simulink model "Virtual_Exhaust_Aftertreatment_Controller_PRT"  (R2016b)
settings: Solver=FixedStepAuto  StartTime=0.0  StopTime=inf  FixedStep=VirtExhATCtrlr.tiSimnTiStep_C  RelTol=1e-3  SampleTimeConstraint=STIndependent  EnableMultiTasking=on
undefined symbols (not defined in the file or in its folder): CAL, SOUIT, T3LIMCL_COEOM_MSK_SY, T3LimCL_stMskEOM1_C, T3LimCL_stMskEOM2_C, T3LimCL_stMskEOM3_C, VirtExhATCtrlr_numHrznSize_CA
libraries: simulink x4
(part 5 of 5)

== system Virtual_Exhaust_Aftertreatment_Controller_PRT/UCatCtrl/Urea_Dosing_Control/Feedback Control/PIDctrl/SAT2 ==
  up : Inport
  u : Inport  Port=2
  lo : Inport  Port=3
  Data Type Duplicate : DataTypeDuplicate  DisableCoverage=on
  Data Type Propagation : S-Function  FunctionName=sfix_dtprop  Parameters=14,PropDataTypeMode,(getdatatypespecs(PropDataType,PropScaling,DblOver,0, 0, PropDataTypeMode, PropScalingMode)),IfRefDouble,IfRefSingle,IsSigned,NumBitsBase,NumBitsMult,NumBitsAdd,(sort(reshape(round(NumBitsAllowFinal), prod(size(NumBitsAllowFinal)),1))),PropScalingMode,ValuesUsedBestPrec,SlopeBase,SlopeMult,SlopeAdd,BiasBase,BiasMult,BiasAdd,DblOver  SFunctionDeploymentMode=off  EnableBusSupport=off  mask(Data Type Propagation){PropDataTypeMode=Inherit via propagation rule, PropDataType=fixdt(1, 16), IfRefDouble=double, IfRefSingle=single, IsSigned=IsSigned1, NumBitsBase=NumBits1, NumBitsMult=1, NumBitsAdd=0, NumBitsAllowFinal=1:128, PropScalingMode=Inherit via propagation rule, PropScaling=2^-10, ValuesUsedBestPrec=[5 -7], SlopeBase=Slope1, SlopeMult=1, SlopeAdd=0, BiasBase=Bias1, BiasMult=1, BiasAdd=0}
      mask prompts: PropDataTypeMode "Simulink:masks:x1PropagatedDataType_MP"; PropDataType "Simulink:masks:x11PropagatedDataTypeegFixdt116Fixdtsingle_MP"; IfRefDouble "Simulink:masks:x11IfAnyReferenceInputIsDoubleOutputIs_MP"; IfRefSingle "Simulink:masks:x12IfAnyReferenceInputIsSingleOutputIs_MP"; IsSigned "Simulink:masks:x13IsSigned_MP"; NumBitsBase "Simulink:masks:x141NumberofBitsBase_MP"; NumBitsMult "Simulink:masks:x142NumberofBitsMultiplicativeAdjustment_MP"; NumBitsAdd "Simulink:masks:x143NumberofBitsAdditiveAdjustment_MP"; NumBitsAllowFinal "Simulink:masks:x144NumberofBitsAllowableFinalValues_MP"; PropScalingMode "Simulink:masks:x2PropagatedScaling_MP"; PropScaling "Simulink:masks:x21PropagatedScalingSlopeEg29OrSlopeBiasEg1253_MP"; ValuesUsedBestPrec "Simulink:masks:x21ValuesUsedToDetermineBestPrecisionScaling_MP"; SlopeBase "Simulink:masks:x211SlopeBase_MP"; SlopeMult "Simulink:masks:x212SlopeMultiplicativeAdjustment_MP"; SlopeAdd "Simulink:masks:x213SlopeAdditiveAdjustment_MP"; BiasBase "Simulink:masks:x221BiasBase_MP"; BiasMult "Simulink:masks:x222BiasMultiplicativeAdjustment_MP"; BiasAdd "Simulink:masks:x223BiasAdditiveAdjustment_MP"
      mask help: Simulink:masks:DataTypePropagation_MD
      mask init:
      | DblOver = 0;
      mask TypeOptions PropDataTypeMode: Simulink:masks:SpecifyViaDialog | Simulink:masks:InheritViaPropagationRule
      mask Callback PropDataTypeMode: fixptdialog(gcbh)
      mask Callback PropDataType: fixptdialog(gcbh)
      mask TypeOptions IfRefDouble: Simulink:masks:double | Simulink:masks:single
      mask TypeOptions IfRefSingle: Simulink:masks:double | Simulink:masks:single
      mask TypeOptions IsSigned: Simulink:masks:IsSigned1 | Simulink:masks:IsSigned2 | Simulink:masks:IsSigned1OrIsSigned2 | Simulink:masks:TRUE | Simulink:masks:FALSE
      mask TypeOptions NumBitsBase: NumBits1 | NumBits2 | max([NumBits1 NumBits2]) | min([NumBits1 NumBits2]) | NumBits1+NumBits2
      mask TypeOptions PropScalingMode: Simulink:masks:SpecifyViaDialog | Simulink:masks:InheritViaPropagationRule | Simulink:masks:ObtainViaBestPrecision
      mask Callback PropScalingMode: fixptdialog(gcbh)
      mask TypeOptions SlopeBase: Slope1 | Slope2 | max([Slope1 Slope2]) | min([Slope1 Slope2]) | Slope1*Slope2 | Slope1/Slope2 | PosRange1 | PosRange2 | max([PosRange1 PosRange2]) | min([PosRange1 PosRange2]) | PosRange1*PosRange2 | PosRange1/PosRange2
      mask TypeOptions BiasBase: Bias1 | Bias2 | max([Bias1 Bias2]) | min([Bias1 Bias2]) | Bias1*Bias2 | Bias1/Bias2 | Bias1+Bias2 | Bias1-Bias2
      mask Display:
      | port_label('Input',1,'Ref1');
      | port_label('Input',2,'Ref2');
      | port_label('Input',3,'Prop');
  LowerRelop1 : RelationalOperator  DisableCoverage=on  Operator=>  OutDataTypeStr=boolean  RndMeth=Nearest
  Switch : Switch  Criteria=u2 ~= 0  OutDataTypeStr=Inherit: Inherit via back propagation  ZeroCross=off
  Switch2 : Switch  Criteria=u2 ~= 0  OutMin=OutMin  OutMax=OutMax  OutDataTypeStr=Inherit: Inherit via back propagation  ZeroCross=off
  UpperRelop : RelationalOperator  DisableCoverage=on  Operator=<  OutDataTypeStr=boolean  RndMeth=Nearest
  y : Outport  OutMin=OutMin  OutMax=OutMax
  wires:
  up/1 -> Switch2/1, LowerRelop1/2
  u/1 -> Data Type Propagation/2, Data Type Propagation/1, LowerRelop1/1, Switch/3, UpperRelop/1
  lo/1 -> Switch/1, UpperRelop/2
  Switch/1 -> Data Type Duplicate/2, Switch2/3, Data Type Propagation/3
  Switch2/1 -> Data Type Duplicate/1, y/1
  LowerRelop1/1 -> Switch2/2
  UpperRelop/1 -> Switch/2

== system Virtual_Exhaust_Aftertreatment_Controller_PRT/UCatCtrl/Urea_Dosing_Control/Feedback Control/PIDctrl/Subsystem ==
  X : Inport
  Ki : Inport  Port=2
  Reset : Inport  Port=3
  Y0_YReset : Inport  Port=4
  Min : Inport  Port=5
  Max : Inport  Port=6
  dT : Inport  Port=7
  Add1 : Sum
  Add2 : Sum
  AntiWindUp : Subsystem
  Constant2 : Constant  Value=0  SampleTime=-1
  Constant3 : Constant  Value=0  SampleTime=-1
  Kp = 0 : Constant  Value=0  SampleTime=-1
  Product1 : Product  RndMeth=Zero
  Product2 : Product  RndMeth=Zero
  Product3 : Product  RndMeth=Zero
  Saturation : Subsystem
  Switch1 : Switch  Criteria=u2 ~= 0
  Switch2 : Switch  Criteria=u2 ~= 0
  Switch3 : Switch  Criteria=u2 ~= 0
  Unit Delay External IC : Subsystem  mask(Unit Delay External Initial Condition){tsamp=-1}
      mask prompts: tsamp "Simulink:masks:SampleTime_MP"
      mask help: Simulink:masks:UnitDelayExternalInitialCondition_MD
      mask Display: dpoly(1,[1 0],'z')
  Unit Delay External IC1 : Subsystem  mask(Unit Delay External Initial Condition){tsamp=-1}
      mask prompts: tsamp "Simulink:masks:SampleTime_MP"
      mask help: Simulink:masks:UnitDelayExternalInitialCondition_MD
      mask Display: dpoly(1,[1 0],'z')
  Y : Outport
  wires:
  Constant3/1 -> Switch3/1
  AntiWindUp/1(Clamp) -> Switch1/2
  Saturation/1(Y) -> Unit Delay External IC1/1(u)
  Product1/1 -> Switch3/3
  Product2/1 -> Product3/1
  Product3/1 -> AntiWindUp/1(PreInteg), Switch1/3
  Add1/1 -> Switch2/3
  Saturation/2(Sat) -> AntiWindUp/2(Sat)
  Switch1/1 -> Add1/1
  Switch3/1 -> Add2/1
  Add2/1 -> Saturation/2(X)
  Switch2/1 -> Add2/2, Unit Delay External IC/1(u)
  Reset/1 -> Switch2/2, Switch3/2
  X/1 -> Product2/1, Product1/1
  Max/1 -> Saturation/1(Max)
  Y0_YReset/1 -> Switch2/1, Unit Delay External IC/2(IC), Unit Delay External IC1/2(IC)
  Unit Delay External IC1/1(y) -> Y/1
  dT/1 -> Product3/2
  Unit Delay External IC/1(y) -> Add1/2
  Ki/1 -> Product2/2
  Min/1 -> Saturation/3(Min)
  Kp = 0/1 -> Product1/2
  Constant2/1 -> Switch1/1

== system Virtual_Exhaust_Aftertreatment_Controller_PRT/UCatCtrl/Urea_Dosing_Control/Feedback Control/PIDctrl/Subsystem1 ==
  note: ( U(k) - U(k-1) )
  note: U(k)
  X : Inport
  Y0 : Inport  Port=2
  dT : Inport  Port=3
  Divide : Product  Inputs=*/
  Subtract : Sum  Inputs=+-
  Unit Delay External IC : Subsystem  mask(Unit Delay External Initial Condition){tsamp=-1}
      mask prompts: tsamp "Simulink:masks:SampleTime_MP"
      mask help: Simulink:masks:UnitDelayExternalInitialCondition_MD
      mask Display: dpoly(1,[1 0],'z')
  Y : Outport
  wires:
  X/1 -> Divide/1
  Divide/1 -> Subtract/1, Unit Delay External IC/1(u)
  dT/1 -> Divide/2
  Subtract/1 -> Y/1
  Unit Delay External IC/1(y) -> Subtract/2  "U(k-1)"
  Y0/1 -> Unit Delay External IC/2(IC)  "XX"

== system Virtual_Exhaust_Aftertreatment_Controller_PRT/UCatCtrl/Urea_Dosing_Control/Feedback Control/PIDctrl/Subsystem2 ==
  X : Inport
  Ki : Inport  Port=2
  Reset : Inport  Port=3
  Y0_YReset : Inport  Port=4
  Min : Inport  Port=5
  Max : Inport  Port=6
  dT : Inport  Port=7
  Add1 : Sum
  Add2 : Sum
  AntiWindUp : Subsystem
  Constant2 : Constant  Value=0  SampleTime=-1
  Constant3 : Constant  Value=0  SampleTime=-1
  Kp = 0 : Constant  Value=0  SampleTime=-1
  Product1 : Product  RndMeth=Zero
  Product2 : Product  RndMeth=Zero
  Product3 : Product  RndMeth=Zero
  Saturation : Subsystem
  Switch1 : Switch  Criteria=u2 ~= 0
  Switch2 : Switch  Criteria=u2 ~= 0
  Switch3 : Switch  Criteria=u2 ~= 0
  Unit Delay External IC : Subsystem  mask(Unit Delay External Initial Condition){tsamp=-1}
      mask prompts: tsamp "Simulink:masks:SampleTime_MP"
      mask help: Simulink:masks:UnitDelayExternalInitialCondition_MD
      mask Display: dpoly(1,[1 0],'z')
  Unit Delay External IC1 : Subsystem  mask(Unit Delay External Initial Condition){tsamp=-1}
      mask prompts: tsamp "Simulink:masks:SampleTime_MP"
      mask help: Simulink:masks:UnitDelayExternalInitialCondition_MD
      mask Display: dpoly(1,[1 0],'z')
  Y : Outport
  wires:
  Constant2/1 -> Switch1/1
  Kp = 0/1 -> Product1/2
  Min/1 -> Saturation/3(Min)
  Ki/1 -> Product2/2
  Unit Delay External IC/1(y) -> Add1/2
  dT/1 -> Product3/2
  Unit Delay External IC1/1(y) -> Y/1
  Y0_YReset/1 -> Unit Delay External IC1/2(IC), Unit Delay External IC/2(IC), Switch2/1
  Max/1 -> Saturation/1(Max)
  X/1 -> Product1/1, Product2/1
  Reset/1 -> Switch3/2, Switch2/2
  Switch2/1 -> Unit Delay External IC/1(u), Add2/2
  Add2/1 -> Saturation/2(X)
  Switch3/1 -> Add2/1
  Switch1/1 -> Add1/1
  Saturation/2(Sat) -> AntiWindUp/2(Sat)
  Add1/1 -> Switch2/3
  Product3/1 -> Switch1/3, AntiWindUp/1(PreInteg)
  Product2/1 -> Product3/1
  Product1/1 -> Switch3/3
  Saturation/1(Y) -> Unit Delay External IC1/1(u)
  AntiWindUp/1(Clamp) -> Switch1/2
  Constant3/1 -> Switch3/1

== system Virtual_Exhaust_Aftertreatment_Controller_PRT/UCatCtrl/SCR_Prediction/Main/UCat NH3 Load Prediction/Discrete Integrator/AntiWindUp ==
  PreInteg : Inport
  Sat : Inport  Port=2
  Constant1 : Constant  Value=0  SampleTime=-1
  Logical1 : Logic  AllPortsSameDT=off  OutDataTypeStr=boolean
  Relational1 : RelationalOperator  Operator===  OutDataTypeStr=boolean  RndMeth=Nearest
  Relational2 : RelationalOperator  Operator=~=  OutDataTypeStr=boolean  RndMeth=Nearest
  Sign1 : Signum
  UnitDelay2 : UnitDelay  SampleTime=-1
  Clamp : Outport
  wires:
  PreInteg/1 -> Sign1/1
  Sign1/1 -> Relational1/1
  Relational1/1 -> Logical1/1
  Sat/1 -> UnitDelay2/1
  Logical1/1 -> Clamp/1
  UnitDelay2/1 -> Relational2/1, Relational1/2
  Relational2/1 -> Logical1/2
  Constant1/1 -> Relational2/2

== system Virtual_Exhaust_Aftertreatment_Controller_PRT/UCatCtrl/SCR_Prediction/Main/UCat NH3 Load Prediction/Discrete Integrator/Saturation ==
  Max : Inport
  X : Inport  Port=2
  Min : Inport  Port=3
  Constant1 : Constant  SampleTime=-1
  Constant2 : Constant  Value=-1  SampleTime=-1
  Constant3 : Constant  Value=0  SampleTime=-1
  Relational1 : RelationalOperator  Operator=<  OutDataTypeStr=boolean  RndMeth=Nearest
  Relational2 : RelationalOperator  Operator=>  OutDataTypeStr=boolean  RndMeth=Nearest
  Switch{1..4} (4 alike) : Switch  Criteria=u2 ~= 0
  Y : Outport
  Sat : Outport  Port=2
  wires:
  Relational1/1 -> Switch4/2, Switch2/2
  Max/1 -> Switch2/1, Relational1/1
  Relational2/1 -> Switch3/2, Switch1/2
  Min/1 -> Relational2/1, Switch1/1
  Switch1/1 -> Switch2/3
  X/1 -> Relational1/2, Relational2/2, Switch1/3
  Switch2/1 -> Y/1
  Constant1/1 -> Switch4/1
  Switch3/1 -> Switch4/3
  Switch4/1 -> Sat/1
  Constant2/1 -> Switch3/1
  Constant3/1 -> Switch3/3

== system Virtual_Exhaust_Aftertreatment_Controller_PRT/UCatCtrl/SCR_Prediction/Main/UCat NH3 Load Prediction/Discrete Integrator/Unit Delay External IC ==
  note: Xnew
  note: Initial Value
  u : Inport
  IC : Inport  Port=2
  FixPt Constant : Constant  DisableCoverage=on  Value=0  OutDataTypeStr=fixdt(0,8,0)  SampleTime=-1
  FixPt Data Type Duplicate1 : DataTypeDuplicate  DisableCoverage=on  NumInputPorts=3
  FixPt Unit Delay1 : UnitDelay  DisableCoverage=on  InitialCondition=0.0  SampleTime=tsamp  HasFrameUpgradeWarning=off
  FixPt Unit Delay2 : UnitDelay  DisableCoverage=on  InitialCondition=1  SampleTime=tsamp
  Init : Switch  Criteria=u2 ~= 0  OutDataTypeStr=Inherit: Inherit via back propagation  ZeroCross=off
  y : Outport
  wires:
  FixPt Unit Delay1/1 -> Init/3  "Xold"
  Init/1 -> y/1, FixPt Data Type Duplicate1/1
  FixPt Unit Delay2/1 -> Init/2
  FixPt Constant/1 -> FixPt Unit Delay2/1
  u/1 -> FixPt Unit Delay1/1, FixPt Data Type Duplicate1/2
  IC/1 -> Init/1, FixPt Data Type Duplicate1/3

== system Virtual_Exhaust_Aftertreatment_Controller_PRT/UCatCtrl/SCR_Prediction/Main/UCat NH3 Load Prediction/Discrete Integrator/Unit Delay External IC1 ==
  note: Xnew
  note: Initial Value
  u : Inport
  IC : Inport  Port=2
  FixPt Constant : Constant  DisableCoverage=on  Value=0  OutDataTypeStr=fixdt(0,8,0)  SampleTime=-1
  FixPt Data Type Duplicate1 : DataTypeDuplicate  DisableCoverage=on  NumInputPorts=3
  FixPt Unit Delay1 : UnitDelay  DisableCoverage=on  InitialCondition=0.0  SampleTime=tsamp  HasFrameUpgradeWarning=off
  FixPt Unit Delay2 : UnitDelay  DisableCoverage=on  InitialCondition=1  SampleTime=tsamp
  Init : Switch  Criteria=u2 ~= 0  OutDataTypeStr=Inherit: Inherit via back propagation  ZeroCross=off
  y : Outport
  wires:
  FixPt Unit Delay1/1 -> Init/3  "Xold"
  Init/1 -> y/1, FixPt Data Type Duplicate1/1
  FixPt Unit Delay2/1 -> Init/2
  FixPt Constant/1 -> FixPt Unit Delay2/1
  u/1 -> FixPt Unit Delay1/1, FixPt Data Type Duplicate1/2
  IC/1 -> Init/1, FixPt Data Type Duplicate1/3

== system Virtual_Exhaust_Aftertreatment_Controller_PRT/UCatCtrl/SCR_Prediction/Main/UCat NH3 Load Prediction/GOTO_ATS_mflNH3OxiUCatUs_mgps/GainXX ==
  In : Inport
  Out : Outport
  wires:
  In/1 -> Out/1

== system Virtual_Exhaust_Aftertreatment_Controller_PRT/UCatCtrl/SCR_Prediction/Main/UCat NH3 Load Prediction/NH3 Oxidation/NH3 Oxidation ==
  ATS_mEstNH3LdUCat : Inport
  ATS_tEstUCatAvrg : Inport  Port=2
  ATS_rNH3Curr_ppm : Inport  Port=3
  "ATS_mflEG " : Inport  Port=4
  ATS_facEffUCatAge : Inport  Port=5
  Constant1 : Constant  Value=1000  SampleTime=-1
  Constant2 : Constant  Value=0  SampleTime=-1
  Constant6 : Constant  SampleTime=-1
  Lookup_n-D_3 : Lookup_n-D  BreakpointsForDimension1=[100;150;200;250;300;350;400;450;500;550;700;1000]  BreakpointsForDimension2=[0 1.89999997615814 3.79999995231628 5.69999980926514 7.59999990463257 11.3999996185303 15.1999998092651 26.6000003814697]  Table=[0 3.70879998570075e-20 7.42519969327932e-20 1.10959997771212e-19 1.48200004990473e-19 2.22679993579601e-19 2.97160008018124e-19 5.19840001597725e-19;0 9.04399990686384e-18 1.81639995140478e-17 2.72839999484124e-17 3.6404000382777e-17 5.45679998968249e-17 7.28080007655541e-17 1.26919999151736e-16;0 6.97680021648363e-16 1.39840004454442e-15 2.09000001075784e-15 2.78920008596961e-15 4.18760002463491e-15 5.57840017193921e-15 9.72799975746145e-15;0 2.3332000258702e-14 4.66640005174039e-14 6.99959973879741e-14 9.34799994031267e-14 1.39840003183893e-13 1.86200000188395e-13 3.26040003372288e-13;0 4.22559990470584e-13 8.43599983705451e-13 1.26920002285758e-12 1.6871999674109e-12 2.53840004571515e-12 3.38199997521049e-12 5.91280019737739e-12;0 4.81080019570923e-12 9.57599971540546e-12 1.43639995731082e-11 1.92279994010169e-11 2.88040008511459e-11 3.84559988020339e-11 6.73359978886623e-11;0 3.81519989212098e-11 7.59999979615955e-11 1.13999996942393e-10 1.51999995923191e-10 2.28759997056294e-10 3.04759995017889e-10 5.33520005951971e-10;0 2.2648000141956e-10 4.53720006010627e-10 6.80960010601694e-10 9.04399999335226e-10 1.36040001486038e-09 1.81640003038552e-09 3.17679993422359e-09;0 1.07160003093298e-09 2.14320006186597e-09 3.22239990246942e-09 4.2939998223801e-09 6.43720010629067e-09 8.5879996447602e-09 1.49720005282461e-08;0 4.20279988588845e-09 8.35999980353108e-09 1.26159998004027e-08 1.67959992580791e-08 2.52319996008055e-08 3.35919985161581e-08 5.88239998933204e-08;0 1.08679998334083e-07 2.16600000157996e-07 3.25280012702933e-07 4.3471999333633e-07 6.51320021916035e-07 8.66400000631984e-07 1.51999995523511e-06;0 7.28080021872302e-06 1.45920002978528e-05 2.18120003410149e-05 2.91079995804466e-05 4.37000016972888e-05 5.82159991608933e-05 0.000101839999842923]  ExtrapMethod=Clip  UseLastTableValue=on  RndMeth=Simplest  InputSameDT=on
  Lookup_n-D_4 : Lookup_n-D  BreakpointsForDimension1=[0;0.100000001490116;0.200000002980232;0.300000011920929;0.5;0.75;1]  BreakpointsForDimension2=[0 500 1000 1500 2000 2500 3000]  Table=[0.184162065386772 0.184162065386772 0.184162065386772 0.184162065386772 0.184162065386772 0.184162065386772 0.184162065386772;0.184162065386772 0.184162065386772 0.184162065386772 0.184162065386772 0.184162065386772 0.184162065386772 0.184162065386772;0.184162065386772 0.184162065386772 0.184162065386772 0.184162065386772 0.184162065386772 0.184162065386772 0.184162065386772;0.184162065386772 0.184162065386772 0.184162065386772 0.184162065386772 0.184162065386772 0.184162065386772 0.184162065386772;0.184162065386772 0.184162065386772 0.184162065386772 0.184162065386772 0.184162065386772 0.184162065386772 0.184162065386772;0.184162065386772 0.184162065386772 0.184162065386772 0.184162065386772 0.184162065386772 0.184162065386772 0.184162065386772;0.184162065386772 0.184162065386772 0.184162065386772 0.184162065386772 0.184162065386772 0.184162065386772 0.184162065386772]  RndMeth=Simplest  InputSameDT=on
  Lookup_n-D_5 : Lookup_n-D  BreakpointsForDimension1=[100;150;200;250;300;350;400;450;500;550;700;1000]  BreakpointsForDimension2=[0 75 175 350 550 1000]  Table=[10000000000 10000000000 10000000000 10000000000 10000000000 10000000000;10000000000 10000000000 10000000000 10000000000 10000000000 10000000000;10000000000 10000000000 10000000000 10000000000 10000000000 10000000000;2000000000 2000000000 4499999744 5470000128 12199999488 12199999488;600000000 600000000 1500000000 3100000000 4600000000 4600000000;120000000 120000000 200000000 300000000 450000000 500000000;25000000 25000000 32500000 49000000 51500000 51500000;12000000 12000000 20000000 30000000 38000000 38000000;3500000 3500000 6000000 11500000 14000000 14000000;2500000 2500000 5500000 8500000 10000000 10000000;2000000 2000000 4000000 5000000 8000000 8000000;1000000 1000000 2000000 3000000 5900000 5000000]  RndMeth=Simplest  InputSameDT=on
  Lookup_n-D_6 : Lookup_n-D  Description=output: mg/s  BreakpointsForDimension1=[0;0.100000001490116;0.200000002980232;0.300000011920929;0.5;0.75;1]  BreakpointsForDimension2=[0 500 1000 1500 2000 2500 3000]  Table=[1 1 1 1 1 1 1;1 1 1 1 1 1 1;1 1 1 1 1 1 1;1 1 1 1 1 1 1;1 1 1 1 1 1 1;1 1 1 1 1 1 1;1 1 1 1 1 1 1]  ExtrapMethod=Clip  UseLastTableValue=on  RndMeth=Simplest  InputSameDT=on
  MinMax : MinMax  Function=max  Inputs=2
  rox_gps{,1..3} (4 alike) : Product  SaturateOnIntegerOverflow=on  OutDataTypeStr=Inherit: Same as first input
  ATS_mflNH3OxiUCatUs_mgps : Outport
  wires:
  Lookup_n-D_5/1 -> rox_gps/2
  MinMax/1 -> rox_gps/1
  Constant2/1 -> MinMax/1
  ATS_rNH3Curr_ppm/1 -> Lookup_n-D_5/2
  Lookup_n-D_3/1 -> MinMax/2
  ATS_mEstNH3LdUCat/1 -> Lookup_n-D_3/2
  ATS_tEstUCatAvrg/1 -> Lookup_n-D_3/1, Lookup_n-D_5/1
  rox_gps1/1 -> rox_gps2/1
  Lookup_n-D_4/1 -> rox_gps1/2
  ATS_facEffUCatAge/1 -> Lookup_n-D_4/1
  "ATS_mflEG "/1 -> Lookup_n-D_6/2, Lookup_n-D_4/2
  rox_gps/1 -> rox_gps3/1
  Constant6/1 -> Lookup_n-D_6/1
  Lookup_n-D_6/1 -> rox_gps2/2
  rox_gps2/1 -> ATS_mflNH3OxiUCatUs_mgps/1
  Constant1/1 -> rox_gps3/2
  rox_gps3/1 -> rox_gps1/1

== system Virtual_Exhaust_Aftertreatment_Controller_PRT/UCatCtrl/SCR_Prediction/Main/UCat NH3 Load Prediction/NH3 Oxidation/mg//s to ppm ==
  ATS_mflNH3MetAdapDes_mgps : Inport
  ATS_mflEG : Inport  Port=2
  Divide : Product  Inputs=*/
  Divide1 : Product  Inputs=*/
  MinMax : MinMax  Function=max  Inputs=2
  Product : Product  Inputs=3  RndMeth=Zero
  one1 : Constant  Value=0  SampleTime=-1
  one3 : Constant  Value=3600  SampleTime=-1
  one4 : Constant  Value=29  SampleTime=-1
  one5 : Constant  Value=17  SampleTime=-1
  ATS_rNH3Curr_ppm : Outport
  wires:
  ATS_mflNH3MetAdapDes_mgps/1 -> Product/1
  ATS_mflEG/1 -> MinMax/1
  one3/1 -> Product/2
  one4/1 -> Product/3
  Product/1 -> Divide/1
  one5/1 -> Divide/2
  Divide/1 -> Divide1/1
  Divide1/1 -> ATS_rNH3Curr_ppm/1
  one1/1 -> MinMax/2
  MinMax/1 -> Divide1/2

== system Virtual_Exhaust_Aftertreatment_Controller_PRT/UCatCtrl/SCR_Prediction/Main/UCat Temperature Prediction/DOC Temperature Estimation 1/Calc HeatCapacities ==
  dmEG : Inport
  cpCatBrick : Inport  Port=2
  facVelDpnCor : Inport  Port=3
  cpEGBrick : Inport  Port=4
  mBrick : Inport  Port=5
  arEchExtBrick : Inport  Port=6
  Add1 : Sum  Inputs=+++
  Constant1 : Constant  Value=3.6  SampleTime=-1
  Constant_2 : Constant  Value=0.02  SampleTime=-1
  gainTamb1 : Product  Inputs=*/  SaturateOnIntegerOverflow=on  InputSameDT=on  OutDataTypeStr=Inherit: Same as first input
  gainTamb2 : Product  Inputs=**  SaturateOnIntegerOverflow=on  InputSameDT=on  OutDataTypeStr=Inherit: Same as first input
  gainTamb3 : Product  Inputs=***  SaturateOnIntegerOverflow=on  InputSameDT=on  OutDataTypeStr=Inherit: Same as first input
  gainTamb4 : Product  Inputs=***  SaturateOnIntegerOverflow=on  InputSameDT=on  OutDataTypeStr=Inherit: Same as first input
  cBrick : Outport
  cBrickSum : Outport  Port=2
  cEGBrick : Outport  Port=3
  cBrickEnv : Outport  Port=4
  wires:
  cpCatBrick/1 -> gainTamb2/1
  mBrick/1 -> gainTamb2/2
  dmEG/1 -> gainTamb1/1
  Constant1/1 -> gainTamb1/2
  gainTamb1/1 -> gainTamb3/1
  cpEGBrick/1 -> gainTamb3/2
  Constant_2/1 -> gainTamb3/3, gainTamb4/1
  facVelDpnCor/1 -> gainTamb4/2
  arEchExtBrick/1 -> gainTamb4/3
  gainTamb3/1 -> Add1/2, cEGBrick/1
  gainTamb4/1 -> cBrickEnv/1, Add1/3
  gainTamb2/1 -> Add1/1, cBrick/1
  Add1/1 -> cBrickSum/1

== system Virtual_Exhaust_Aftertreatment_Controller_PRT/UCatCtrl/SCR_Prediction/Main/UCat Temperature Prediction/DOC Temperature Estimation 2/Calc HeatCapacities ==
  dmEG : Inport
  cpCatBrick : Inport  Port=2
  facVelDpnCor : Inport  Port=3
  cpEGBrick : Inport  Port=4
  mBrick : Inport  Port=5
  arEchExtBrick : Inport  Port=6
  Add1 : Sum  Inputs=+++
  Constant1 : Constant  Value=3.6  SampleTime=-1
  Constant_5 : Constant  Value=0.02  SampleTime=-1
  gainTamb1 : Product  Inputs=*/  SaturateOnIntegerOverflow=on  InputSameDT=on  OutDataTypeStr=Inherit: Same as first input
  gainTamb2 : Product  Inputs=**  SaturateOnIntegerOverflow=on  InputSameDT=on  OutDataTypeStr=Inherit: Same as first input
  gainTamb3 : Product  Inputs=***  SaturateOnIntegerOverflow=on  InputSameDT=on  OutDataTypeStr=Inherit: Same as first input
  gainTamb4 : Product  Inputs=***  SaturateOnIntegerOverflow=on  InputSameDT=on  OutDataTypeStr=Inherit: Same as first input
  cBrick : Outport
  cBrickSum : Outport  Port=2
  cEGBrick : Outport  Port=3
  cBrickEnv : Outport  Port=4
  wires:
  cpCatBrick/1 -> gainTamb2/1
  mBrick/1 -> gainTamb2/2
  dmEG/1 -> gainTamb1/1
  Constant1/1 -> gainTamb1/2
  gainTamb1/1 -> gainTamb3/1
  cpEGBrick/1 -> gainTamb3/2
  Constant_5/1 -> gainTamb3/3, gainTamb4/1
  facVelDpnCor/1 -> gainTamb4/2
  arEchExtBrick/1 -> gainTamb4/3
  gainTamb3/1 -> Add1/2, cEGBrick/1
  gainTamb4/1 -> cBrickEnv/1, Add1/3
  gainTamb2/1 -> Add1/1, cBrick/1
  Add1/1 -> cBrickSum/1

== system Virtual_Exhaust_Aftertreatment_Controller_PRT/UCatCtrl/SCR_Prediction/Main/UCat Temperature Prediction/DOC Temperature Estimation 3/Calc HeatCapacities ==
  dmEG : Inport
  cpCatBrick : Inport  Port=2
  facVelDpnCor : Inport  Port=3
  cpEGBrick : Inport  Port=4
  mBrick : Inport  Port=5
  arEchExtBrick : Inport  Port=6
  Add1 : Sum  Inputs=+++
  Constant1 : Constant  Value=3.6  SampleTime=-1
  Constant_8 : Constant  Value=0.02  SampleTime=-1
  gainTamb1 : Product  Inputs=*/  SaturateOnIntegerOverflow=on  InputSameDT=on  OutDataTypeStr=Inherit: Same as first input
  gainTamb2 : Product  Inputs=**  SaturateOnIntegerOverflow=on  InputSameDT=on  OutDataTypeStr=Inherit: Same as first input
  gainTamb3 : Product  Inputs=***  SaturateOnIntegerOverflow=on  InputSameDT=on  OutDataTypeStr=Inherit: Same as first input
  gainTamb4 : Product  Inputs=***  SaturateOnIntegerOverflow=on  InputSameDT=on  OutDataTypeStr=Inherit: Same as first input
  cBrick : Outport
  cBrickSum : Outport  Port=2
  cEGBrick : Outport  Port=3
  cBrickEnv : Outport  Port=4
  wires:
  cpCatBrick/1 -> gainTamb2/1
  mBrick/1 -> gainTamb2/2
  dmEG/1 -> gainTamb1/1
  Constant1/1 -> gainTamb1/2
  gainTamb1/1 -> gainTamb3/1
  cpEGBrick/1 -> gainTamb3/2
  Constant_8/1 -> gainTamb3/3, gainTamb4/1
  facVelDpnCor/1 -> gainTamb4/2
  arEchExtBrick/1 -> gainTamb4/3
  gainTamb3/1 -> Add1/2, cEGBrick/1
  gainTamb4/1 -> cBrickEnv/1, Add1/3
  gainTamb2/1 -> Add1/1, cBrick/1
  Add1/1 -> cBrickSum/1

== system Virtual_Exhaust_Aftertreatment_Controller_PRT/UCatCtrl/SCR_Prediction/Main/UCat Temperature Prediction/DOC Temperature Estimation 4/Calc HeatCapacities ==
  dmEG : Inport
  cpCatBrick : Inport  Port=2
  facVelDpnCor : Inport  Port=3
  cpEGBrick : Inport  Port=4
  mBrick : Inport  Port=5
  arEchExtBrick : Inport  Port=6
  Add1 : Sum  Inputs=+++
  Constant1 : Constant  Value=3.6  SampleTime=-1
  Constant_11 : Constant  Value=0.02  SampleTime=-1
  gainTamb1 : Product  Inputs=*/  SaturateOnIntegerOverflow=on  InputSameDT=on  OutDataTypeStr=Inherit: Same as first input
  gainTamb2 : Product  Inputs=**  SaturateOnIntegerOverflow=on  InputSameDT=on  OutDataTypeStr=Inherit: Same as first input
  gainTamb3 : Product  Inputs=***  SaturateOnIntegerOverflow=on  InputSameDT=on  OutDataTypeStr=Inherit: Same as first input
  gainTamb4 : Product  Inputs=***  SaturateOnIntegerOverflow=on  InputSameDT=on  OutDataTypeStr=Inherit: Same as first input
  cBrick : Outport
  cBrickSum : Outport  Port=2
  cEGBrick : Outport  Port=3
  cBrickEnv : Outport  Port=4
  wires:
  cpCatBrick/1 -> gainTamb2/1
  mBrick/1 -> gainTamb2/2
  dmEG/1 -> gainTamb1/1
  Constant1/1 -> gainTamb1/2
  gainTamb1/1 -> gainTamb3/1
  cpEGBrick/1 -> gainTamb3/2
  Constant_11/1 -> gainTamb3/3, gainTamb4/1
  facVelDpnCor/1 -> gainTamb4/2
  arEchExtBrick/1 -> gainTamb4/3
  gainTamb3/1 -> Add1/2, cEGBrick/1
  gainTamb4/1 -> cBrickEnv/1, Add1/3
  gainTamb2/1 -> Add1/1, cBrick/1
  Add1/1 -> cBrickSum/1

== system Virtual_Exhaust_Aftertreatment_Controller_PRT/UCatCtrl/Urea_Dosing_Control/Dosing Limitation/DepLimCor/ Calc facOpMode_OriginalVersion/Subsystem ==
  stOpModeMsk : Inport
  stOpMode : Inport  Port=2
  Relational Operator : RelationalOperator  Operator===  OutDataTypeStr=boolean  RndMeth=Simplest
  Out : Outport
  wires:
  stOpMode/1 -> Relational Operator/1
  stOpModeMsk/1 -> Relational Operator/2
  Relational Operator/1 -> Out/1

== system Virtual_Exhaust_Aftertreatment_Controller_PRT/UCatCtrl/Urea_Dosing_Control/Dosing Limitation/DepLimCor/ Calc facOpMode_OriginalVersion/Subsystem1 ==
  stOpModeMsk : Inport
  stOpMode : Inport  Port=2
  Relational Operator : RelationalOperator  Operator===  OutDataTypeStr=boolean  RndMeth=Simplest
  Out : Outport
  wires:
  stOpMode/1 -> Relational Operator/1
  stOpModeMsk/1 -> Relational Operator/2
  Relational Operator/1 -> Out/1

== system Virtual_Exhaust_Aftertreatment_Controller_PRT/UCatCtrl/Urea_Dosing_Control/Dosing Limitation/DepLimCor/ Calc facOpMode_OriginalVersion/Subsystem2 ==
  stOpModeMsk : Inport
  stOpMode : Inport  Port=2
  Relational Operator : RelationalOperator  Operator===  OutDataTypeStr=boolean  RndMeth=Simplest
  Out : Outport
  wires:
  stOpMode/1 -> Relational Operator/1
  stOpModeMsk/1 -> Relational Operator/2
  Relational Operator/1 -> Out/1

== system Virtual_Exhaust_Aftertreatment_Controller_PRT/UCatCtrl/Urea_Dosing_Control/Dosing Limitation/DepLimCor/ Calc facOpMode_OriginalVersion/Subsystem3 ==
  stOpModeMsk : Inport
  stOpMode : Inport  Port=2
  Relational Operator : RelationalOperator  Operator===  OutDataTypeStr=boolean  RndMeth=Simplest
  Out : Outport
  wires:
  stOpMode/1 -> Relational Operator/1
  stOpModeMsk/1 -> Relational Operator/2
  Relational Operator/1 -> Out/1

== system Virtual_Exhaust_Aftertreatment_Controller_PRT/UCatCtrl/Urea_Dosing_Control/Dosing Limitation/DepLimCor/ Calc facOpMode_OriginalVersion/T3LimCL_EOMSelection ==
  note: OM1 - PnE
      | OM2- Regen
      | OM3-SCRheatUp
      | Others
  note: T3LIMCL_COEOM_MSK_SY.Value	= 65535;
      | T3LimCL_stMskEOM1_C.Value   = 1048577;
      | T3LimCL_stMskEOM2_C.Value   = 1048576;
      | T3LimCL_stMskEOM3_C.Value   = 1048570;
  CoEOM_stOpModeAct : Inport
  Bitwise Operator_{1..4} (4 alike) : simulink/Logic and Bit Operations/Bitwise Operator  logicop=AND  UseBitMask=off  NumInputPorts=2  BitMask=bin2dec('11011001')  BitMaskRealWorld=Stored Integer
  Constant : Constant  Value=0  OutDataTypeStr=OneToOne_U32
  Constant1 : Constant  Value=T3LIMCL_COEOM_MSK_SY
  Constant2 : Constant  Value=T3LimCL_stMskEOM1_C
  Constant3 : Constant  Value=T3LimCL_stMskEOM2_C
  Constant4 : Constant  Value=T3LimCL_stMskEOM3_C
  Relational Operator_1 : RelationalOperator  Operator=~=  OutDataTypeStr=OneToOne_U8  RndMeth=Nearest
  Relational Operator_2 : RelationalOperator  Operator=~=  OutDataTypeStr=OneToOne_U8  RndMeth=Nearest
  Relational Operator_3 : RelationalOperator  Operator=~=  OutDataTypeStr=OneToOne_U8  RndMeth=Nearest
  T3LimCL_stEOM1_mp : Outport
  T3LimCL_stEOM2_mp : Outport  Port=2
  T3LimCL_stEOM3_mp : Outport  Port=3
  wires:
  Bitwise Operator_4/1 -> Relational Operator_3/1
  Constant/1 -> Relational Operator_3/2, Relational Operator_2/2, Relational Operator_1/2
  Constant4/1 -> Bitwise Operator_4/2
  Relational Operator_3/1 -> T3LimCL_stEOM3_mp/1  "T3LimCL_stEOM3_mp"
  Bitwise Operator_1/1 -> Bitwise Operator_4/1, Bitwise Operator_3/1, Bitwise Operator_2/1
  Constant3/1 -> Bitwise Operator_3/2
  Relational Operator_2/1 -> T3LimCL_stEOM2_mp/1  "T3LimCL_stEOM2_mp"
  Bitwise Operator_3/1 -> Relational Operator_2/1
  Constant1/1 -> Bitwise Operator_1/2
  Relational Operator_1/1 -> T3LimCL_stEOM1_mp/1  "T3LimCL_stEOM1_mp"
  Bitwise Operator_2/1 -> Relational Operator_1/1
  Constant2/1 -> Bitwise Operator_2/2
  CoEOM_stOpModeAct/1 -> Bitwise Operator_1/1

== system Virtual_Exhaust_Aftertreatment_Controller_PRT/UCatCtrl/Urea_Dosing_Control/Feedback Control/PIDctrl/Subsystem/AntiWindUp ==
  PreInteg : Inport
  Sat : Inport  Port=2
  Constant1 : Constant  Value=0  SampleTime=-1
  Logical1 : Logic  AllPortsSameDT=off  OutDataTypeStr=boolean
  Relational1 : RelationalOperator  Operator===  OutDataTypeStr=boolean  RndMeth=Nearest
  Relational2 : RelationalOperator  Operator=~=  OutDataTypeStr=boolean  RndMeth=Nearest
  Sign1 : Signum
  UnitDelay2 : UnitDelay  SampleTime=-1
  Clamp : Outport
  wires:
  PreInteg/1 -> Sign1/1
  Sign1/1 -> Relational1/1
  Relational1/1 -> Logical1/1
  Sat/1 -> UnitDelay2/1
  Logical1/1 -> Clamp/1
  UnitDelay2/1 -> Relational2/1, Relational1/2
  Relational2/1 -> Logical1/2
  Constant1/1 -> Relational2/2

== system Virtual_Exhaust_Aftertreatment_Controller_PRT/UCatCtrl/Urea_Dosing_Control/Feedback Control/PIDctrl/Subsystem/Saturation ==
  Max : Inport
  X : Inport  Port=2
  Min : Inport  Port=3
  Constant1 : Constant  SampleTime=-1
  Constant2 : Constant  Value=-1  SampleTime=-1
  Constant3 : Constant  Value=0  SampleTime=-1
  Relational1 : RelationalOperator  Operator=<  OutDataTypeStr=boolean  RndMeth=Nearest
  Relational2 : RelationalOperator  Operator=>  OutDataTypeStr=boolean  RndMeth=Nearest
  Switch{1..4} (4 alike) : Switch  Criteria=u2 ~= 0
  Y : Outport
  Sat : Outport  Port=2
  wires:
  Relational1/1 -> Switch4/2, Switch2/2
  Max/1 -> Switch2/1, Relational1/1
  Relational2/1 -> Switch3/2, Switch1/2
  Min/1 -> Relational2/1, Switch1/1
  Switch1/1 -> Switch2/3
  X/1 -> Relational1/2, Relational2/2, Switch1/3
  Switch2/1 -> Y/1
  Constant1/1 -> Switch4/1
  Switch3/1 -> Switch4/3
  Switch4/1 -> Sat/1
  Constant2/1 -> Switch3/1
  Constant3/1 -> Switch3/3

== system Virtual_Exhaust_Aftertreatment_Controller_PRT/UCatCtrl/Urea_Dosing_Control/Feedback Control/PIDctrl/Subsystem/Unit Delay External IC ==
  note: Xnew
  note: Initial Value
  u : Inport
  IC : Inport  Port=2
  FixPt Constant : Constant  DisableCoverage=on  Value=0  OutDataTypeStr=fixdt(0,8,0)  SampleTime=-1
  FixPt Data Type Duplicate1 : DataTypeDuplicate  DisableCoverage=on  NumInputPorts=3
  FixPt Unit Delay1 : UnitDelay  DisableCoverage=on  InitialCondition=0.0  SampleTime=tsamp  HasFrameUpgradeWarning=off
  FixPt Unit Delay2 : UnitDelay  DisableCoverage=on  InitialCondition=1  SampleTime=tsamp
  Init : Switch  Criteria=u2 ~= 0  OutDataTypeStr=Inherit: Inherit via back propagation  ZeroCross=off
  y : Outport
  wires:
  FixPt Unit Delay1/1 -> Init/3  "Xold"
  Init/1 -> y/1, FixPt Data Type Duplicate1/1
  FixPt Unit Delay2/1 -> Init/2
  FixPt Constant/1 -> FixPt Unit Delay2/1
  u/1 -> FixPt Unit Delay1/1, FixPt Data Type Duplicate1/2
  IC/1 -> Init/1, FixPt Data Type Duplicate1/3

== system Virtual_Exhaust_Aftertreatment_Controller_PRT/UCatCtrl/Urea_Dosing_Control/Feedback Control/PIDctrl/Subsystem/Unit Delay External IC1 ==
  note: Xnew
  note: Initial Value
  u : Inport
  IC : Inport  Port=2
  FixPt Constant : Constant  DisableCoverage=on  Value=0  OutDataTypeStr=fixdt(0,8,0)  SampleTime=-1
  FixPt Data Type Duplicate1 : DataTypeDuplicate  DisableCoverage=on  NumInputPorts=3
  FixPt Unit Delay1 : UnitDelay  DisableCoverage=on  InitialCondition=0.0  SampleTime=tsamp  HasFrameUpgradeWarning=off
  FixPt Unit Delay2 : UnitDelay  DisableCoverage=on  InitialCondition=1  SampleTime=tsamp
  Init : Switch  Criteria=u2 ~= 0  OutDataTypeStr=Inherit: Inherit via back propagation  ZeroCross=off
  y : Outport
  wires:
  FixPt Unit Delay1/1 -> Init/3  "Xold"
  Init/1 -> y/1, FixPt Data Type Duplicate1/1
  FixPt Unit Delay2/1 -> Init/2
  FixPt Constant/1 -> FixPt Unit Delay2/1
  u/1 -> FixPt Unit Delay1/1, FixPt Data Type Duplicate1/2
  IC/1 -> Init/1, FixPt Data Type Duplicate1/3

== system Virtual_Exhaust_Aftertreatment_Controller_PRT/UCatCtrl/Urea_Dosing_Control/Feedback Control/PIDctrl/Subsystem1/Unit Delay External IC ==
  note: Initial Value
  note: Xnew
  u : Inport
  IC : Inport  Port=2
  FixPt Constant : Constant  DisableCoverage=on  Value=0  OutDataTypeStr=fixdt(0,8,0)
  FixPt Data Type Duplicate1 : DataTypeDuplicate  DisableCoverage=on  NumInputPorts=3
  FixPt Unit Delay1 : UnitDelay  DisableCoverage=on  InitialCondition=0.0  SampleTime=tsamp  HasFrameUpgradeWarning=off
  FixPt Unit Delay2 : UnitDelay  DisableCoverage=on  InitialCondition=1  SampleTime=tsamp
  Init : Switch  Criteria=u2 ~= 0  OutDataTypeStr=Inherit: Inherit via back propagation  ZeroCross=off
  State Control : StateControl  DisableCoverage=on
  y : Outport
  wires:
  IC/1 -> FixPt Data Type Duplicate1/3, Init/1
  u/1 -> FixPt Data Type Duplicate1/2, FixPt Unit Delay1/1
  FixPt Constant/1 -> FixPt Unit Delay2/1
  FixPt Unit Delay2/1 -> Init/2
  Init/1 -> FixPt Data Type Duplicate1/1, y/1
  FixPt Unit Delay1/1 -> Init/3  "Xold"

== system Virtual_Exhaust_Aftertreatment_Controller_PRT/UCatCtrl/Urea_Dosing_Control/Feedback Control/PIDctrl/Subsystem2/AntiWindUp ==
  PreInteg : Inport
  Sat : Inport  Port=2
  Constant1 : Constant  Value=0  SampleTime=-1
  Logical1 : Logic  AllPortsSameDT=off  OutDataTypeStr=boolean
  Relational1 : RelationalOperator  Operator===  OutDataTypeStr=boolean  RndMeth=Nearest
  Relational2 : RelationalOperator  Operator=~=  OutDataTypeStr=boolean  RndMeth=Nearest
  Sign1 : Signum
  UnitDelay2 : UnitDelay  SampleTime=-1
  Clamp : Outport
  wires:
  Constant1/1 -> Relational2/2
  Relational2/1 -> Logical1/2
  UnitDelay2/1 -> Relational1/2, Relational2/1
  Logical1/1 -> Clamp/1
  Sat/1 -> UnitDelay2/1
  Relational1/1 -> Logical1/1
  Sign1/1 -> Relational1/1
  PreInteg/1 -> Sign1/1

== system Virtual_Exhaust_Aftertreatment_Controller_PRT/UCatCtrl/Urea_Dosing_Control/Feedback Control/PIDctrl/Subsystem2/Saturation ==
  Max : Inport
  X : Inport  Port=2
  Min : Inport  Port=3
  Constant1 : Constant  SampleTime=-1
  Constant2 : Constant  Value=-1  SampleTime=-1
  Constant3 : Constant  Value=0  SampleTime=-1
  Relational1 : RelationalOperator  Operator=<  OutDataTypeStr=boolean  RndMeth=Nearest
  Relational2 : RelationalOperator  Operator=>  OutDataTypeStr=boolean  RndMeth=Nearest
  Switch{1..4} (4 alike) : Switch  Criteria=u2 ~= 0
  Y : Outport
  Sat : Outport  Port=2
  wires:
  Constant3/1 -> Switch3/3
  Constant2/1 -> Switch3/1
  Switch4/1 -> Sat/1
  Switch3/1 -> Switch4/3
  Constant1/1 -> Switch4/1
  Switch2/1 -> Y/1
  X/1 -> Switch1/3, Relational2/2, Relational1/2
  Switch1/1 -> Switch2/3
  Min/1 -> Switch1/1, Relational2/1
  Relational2/1 -> Switch1/2, Switch3/2
  Max/1 -> Relational1/1, Switch2/1
  Relational1/1 -> Switch2/2, Switch4/2

== system Virtual_Exhaust_Aftertreatment_Controller_PRT/UCatCtrl/Urea_Dosing_Control/Feedback Control/PIDctrl/Subsystem2/Unit Delay External IC ==
  note: Initial Value
  note: Xnew
  u : Inport
  IC : Inport  Port=2
  FixPt Constant : Constant  DisableCoverage=on  Value=0  OutDataTypeStr=fixdt(0,8,0)  SampleTime=-1
  FixPt Data Type Duplicate1 : DataTypeDuplicate  DisableCoverage=on  NumInputPorts=3
  FixPt Unit Delay1 : UnitDelay  DisableCoverage=on  InitialCondition=0.0  SampleTime=tsamp  HasFrameUpgradeWarning=off
  FixPt Unit Delay2 : UnitDelay  DisableCoverage=on  InitialCondition=1  SampleTime=tsamp
  Init : Switch  Criteria=u2 ~= 0  OutDataTypeStr=Inherit: Inherit via back propagation  ZeroCross=off
  y : Outport
  wires:
  IC/1 -> FixPt Data Type Duplicate1/3, Init/1
  u/1 -> FixPt Data Type Duplicate1/2, FixPt Unit Delay1/1
  FixPt Constant/1 -> FixPt Unit Delay2/1
  FixPt Unit Delay2/1 -> Init/2
  Init/1 -> FixPt Data Type Duplicate1/1, y/1
  FixPt Unit Delay1/1 -> Init/3  "Xold"

== system Virtual_Exhaust_Aftertreatment_Controller_PRT/UCatCtrl/Urea_Dosing_Control/Feedback Control/PIDctrl/Subsystem2/Unit Delay External IC1 ==
  note: Initial Value
  note: Xnew
  u : Inport
  IC : Inport  Port=2
  FixPt Constant : Constant  DisableCoverage=on  Value=0  OutDataTypeStr=fixdt(0,8,0)  SampleTime=-1
  FixPt Data Type Duplicate1 : DataTypeDuplicate  DisableCoverage=on  NumInputPorts=3
  FixPt Unit Delay1 : UnitDelay  DisableCoverage=on  InitialCondition=0.0  SampleTime=tsamp  HasFrameUpgradeWarning=off
  FixPt Unit Delay2 : UnitDelay  DisableCoverage=on  InitialCondition=1  SampleTime=tsamp
  Init : Switch  Criteria=u2 ~= 0  OutDataTypeStr=Inherit: Inherit via back propagation  ZeroCross=off
  y : Outport
  wires:
  IC/1 -> FixPt Data Type Duplicate1/3, Init/1
  u/1 -> FixPt Data Type Duplicate1/2, FixPt Unit Delay1/1
  FixPt Constant/1 -> FixPt Unit Delay2/1
  FixPt Unit Delay2/1 -> Init/2
  Init/1 -> FixPt Data Type Duplicate1/1, y/1
  FixPt Unit Delay1/1 -> Init/3  "Xold"
